simulink model "TD_ALBUQUERQUE_EVANGELISTA"  (R2020a)
settings: Solver=FixedStepAuto  StartTime=0.0  StopTime=tf  FixedStep=Ts  RelTol=1e-3
values from neighbouring files (symbols this model uses):
  alphas = [0 ; pi/2; 0  ; pi/2; -pi/2; pi/2;  0]    [Matlab_model.m]    (also in init.m)
  ds = [0 ;   0 ; d3 ;  0  ;    0 ;   0 ;  0]    [Matlab_model.m]    (also in init.m)
  Gravity = [0;0;-9.81]    [init.m]
  Gs = [G1,G2,G3,G4,G5,G6]    [Matlab_model.m]    (also in init.m)
  I = eye(3)    [Matlab_model.m]    (also in init.m = cat(3, I1,I2,I3,I4,I5,I6))
  Jm = 10e-6.*[1;1;1;1;1;1]    [Matlab_model.m]    (also in init.m)
  Kd = [1000;1000;500;100;100;500]    [init.m]
  Kp = [5000;8000;5500;800;5500;2500]    [init.m]
  m = [m1;m2;m3;m4;m5;m6]    [Matlab_model.m]    (also in init.m)
  Offset = [0; 0; pi/2; 0; 0; 0]    [init.m]
  q_dot_i = [0;0;0;0;0;0]    [Matlab_model.m]    (also in init.m)
  qdf = [0;1;0;0;0;0]    [Matlab_model.m]    (also in init.m)
  qdi = [-1;0;-1;-1;-1;-1]    [Matlab_model.m]    (also in init.m)
  red = [100;100;100;70;70;70]    [Matlab_model.m]    (also in init.m)
  rs = [r1;   0 ; 0  ; r4  ;    0 ;   0 ; rE]    [Matlab_model.m]    (also in init.m)
settings Model: OrderedModelArguments=off  Creator=vitor  LastModifiedBy=joaov

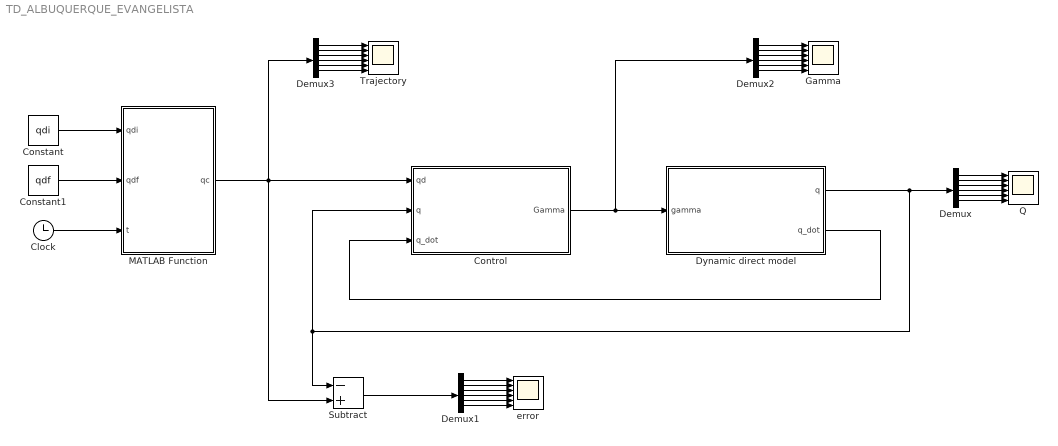
== system TD_ALBUQUERQUE_EVANGELISTA ==
  Clock : Clock
  Constant : Constant  Value=qdi
  Constant1 : Constant  Value=qdf
  Control : Subsystem
  Demux{,1..3} (4 alike) : Demux  Outputs=6
  Dynamic direct model : Subsystem
  Gamma : Scope  NumInputPorts=6
  MATLAB Function : MATLAB Function  TreatAsAtomicUnit=on
  Q : Scope  NumInputPorts=6
  Subtract : Sum  Inputs=-+
  Trajectory : Scope  NumInputPorts=6
  error : Scope  NumInputPorts=6
  wires:
  Demux/2 -> Q/2
  Demux/3 -> Q/3
  Demux/4 -> Q/4
  Demux/5 -> Q/5
  Demux/6 -> Q/6
  Dynamic direct model/1(q) -> Demux/1, Subtract/1, Control/2(q)
  Constant/1 -> MATLAB Function/1(qdi)
  Constant1/1 -> MATLAB Function/2(qdf)
  Clock/1 -> MATLAB Function/3(t)
  Demux1/5 -> error/5
  Demux1/2 -> error/2
  Demux1/3 -> error/3
  Demux1/6 -> error/6
  Demux1/4 -> error/4
  Demux1/1 -> error/1
  Subtract/1 -> Demux1/1
  Demux2/4 -> Gamma/4
  Demux2/2 -> Gamma/2
  Demux2/1 -> Gamma/1
  Demux2/5 -> Gamma/5
  Demux2/3 -> Gamma/3
  Demux2/6 -> Gamma/6
  Demux3/5 -> Trajectory/5
  Demux3/2 -> Trajectory/2
  Demux3/3 -> Trajectory/3
  Demux3/1 -> Trajectory/1
  Demux3/6 -> Trajectory/6
  Demux3/4 -> Trajectory/4
  MATLAB Function/1(qc) -> Subtract/2, Control/1(qd), Demux3/1
  Dynamic direct model/2(q_dot) -> Control/3(q_dot)
  Control/1(Gamma) -> Dynamic direct model/1(gamma), Demux2/1
  Demux/1 -> Q/1

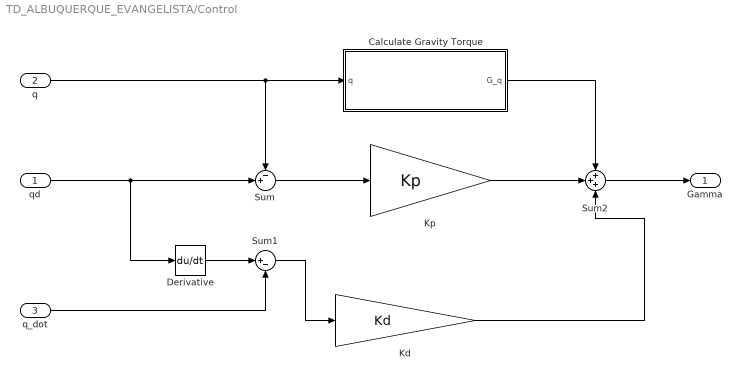
== system TD_ALBUQUERQUE_EVANGELISTA/Control ==
  qd : Inport
  q : Inport  Port=2
  q_dot : Inport  Port=3
  Calculate Gravity Torque : MATLAB Function  TreatAsAtomicUnit=on
  Derivative : Derivative
  Kd : Gain  Gain=Kd
  Kp : Gain  Gain=Kp
  Sum : Sum  Inputs=-+|
  Sum1 : Sum  Inputs=|+-
  Sum2 : Sum  Inputs=+++
  Gamma : Outport
  wires:
  Sum2/1 -> Gamma/1
  Kp/1 -> Sum2/2
  Sum/1 -> Kp/1
  qd/1 -> Sum/2, Derivative/1
  Calculate Gravity Torque/1(G_q) -> Sum2/1
  Kd/1 -> Sum2/3
  Sum1/1 -> Kd/1
  q/1 -> Sum/1, Calculate Gravity Torque/1(q)
  Derivative/1 -> Sum1/1
  q_dot/1 -> Sum1/2

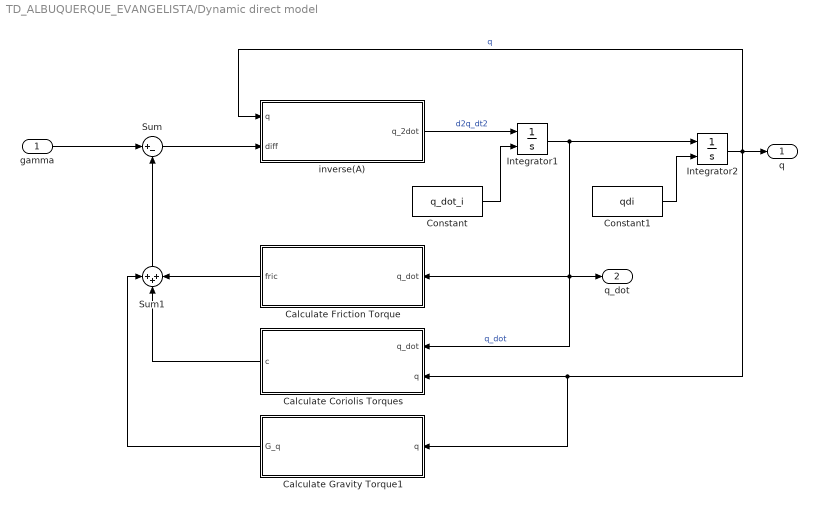
== system TD_ALBUQUERQUE_EVANGELISTA/Dynamic direct model ==
  gamma : Inport
  Calculate Coriolis Torques : MATLAB Function  TreatAsAtomicUnit=on
  Calculate Friction Torque : MATLAB Function  TreatAsAtomicUnit=on
  Calculate Gravity Torque1 : MATLAB Function  TreatAsAtomicUnit=on
  Constant : Constant  Value=q_dot_i
  Constant1 : Constant  Value=qdi
  Integrator1 : Integrator  InitialConditionSource=external
  Integrator2 : Integrator  InitialConditionSource=external
  Sum : Sum  Inputs=|+-
  Sum1 : Sum  Inputs=+++
  inverse(A) : MATLAB Function  TreatAsAtomicUnit=on
  q : Outport
  q_dot : Outport  Port=2
  wires:
  gamma/1 -> Sum/1
  Sum/1 -> inverse(A)/2(diff)
  inverse(A)/1(q_2dot) -> Integrator1/1  "d2q_dt2"
  Integrator1/1 -> Integrator2/1, q_dot/1, Calculate Coriolis Torques/1(q_dot), Calculate Friction Torque/1(q_dot)  "q_dot"
  Integrator2/1 -> Calculate Gravity Torque1/1(q), Calculate Coriolis Torques/2(q), q/1, inverse(A)/1(q)  "q"
  Calculate Coriolis Torques/1(c) -> Sum1/2
  Calculate Gravity Torque1/1(G_q) -> Sum1/1
  Calculate Friction Torque/1(fric) -> Sum1/3
  Sum1/1 -> Sum/2
  Constant/1 -> Integrator1/2
  Constant1/1 -> Integrator2/2

== matlab function TD_ALBUQUERQUE_EVANGELISTA/Dynamic direct model/Calculate Coriolis Torques ==
  data: q_dot input; q input; c output; I parameter; Gs parameter; Offset parameter
function c = ComputeCCTorques(q_dot,q,I,Gs,Offset)
    % Initialisation
    c=zeros(size(q));

    % Paramètres
    iI = I;
    x_G=Gs(1,:)';
    y_G=Gs(2,:)';
    z_G=Gs(3,:)';
    d3 = 0.7; 
    r1 = 0.5; r3=0.0 ; r4 = 0.2;
    alpha = [ 0 , pi/2 , 0 , pi/2 , -pi/2 , pi/2 ] ;
    alpha = [ 0 , pi/2 , 0 , pi/2 , -pi/2 , pi/2 ] ;
    theta = q + Offset;


    % Paramètres relatifs aux corps
    % Axe 1 %[0.80 0 0.05 ; 0 0.80 0 ; 0.05  0  0.10]
    XX1=0.80;
    XY1=0;
    XZ1=0.05;
    YY1=0.80;
    YZ1=0;
    ZZ1=0.10;

    M1=15;

    MX1=0*M1; %x_G1 = 0; y_G1 = 0; z_G1 = -0.25;
    MY1=0*M1;
    MZ1=-0.25*M1;

    % Axe 2 %[0.10  0  0.10; 0  1.50 0 ; 0.10  0  1.50]
    XX2=0.10;
    XY2=0;
    XZ2=0.10;
    YY2=1.50;
    YZ2=0;
    ZZ2=1.50;

    M2=10;

    MX2=0.35*M2; %x_G2 = 0.35; y_G2 = 0; z_G2 = 0;
    MY2=0*M2;
    MZ2=0*M2;

    % Axe 3 %[0.05 0 0 ; 0 0.01 0 ; 0 0 0.05]
    XX3=0.05;
    XY3=0;
    XZ3=0;
    YY3=0.01;
    YZ3=0;
    ZZ3=0.05;

    M3=1;

    MX3=0*M3; %x_G3 = 0; y_G3 = -0.1; z_G3 = 0;
    MY3=-0.1*M3;
    MZ3=0*M3;

    % Axe 4 %[0.50 0 0 ; 0 0.50 0 ; 0 0 0.05]
    XX4=0.50;
    XY4=0;
    XZ4=0;
    YY4=0.50;
    YZ4=0;
    ZZ4=0.05;

    M4=7;

    MX4=0*M4; %x_G4 = 0; y_G4 = 0; z_G4 = 0;
    MY4=0*M4;
    MZ4=0*M4;

    % Axe 5 %[0.01 0 0 ; 0 0.01 0 ; 0 0 0.01]
    XX5=0.01;
    XY5=0;
    XZ5=0;
    YY5=0.01;
    YZ5=0;
    ZZ5=0.01;

    M5=1;

    MX5=0*M5; %x_G5 = 0; y_G5 = 0; z_G5 = 0;
    MY5=0*M5; 
    MZ5=0*M5;

    % Axe 6 %[0.01 0 0 ; 0 0.01 0 ; 0 0 0.01]
    XX6=0.01;
    XY6=0;
    XZ6=0;
    YY6=0.01;
    YZ6=0;
    ZZ6=0.01;

    M6=0.5;

    MX6=0*M6; %x_G6 = 0; y_G6 = 0; z_G6 = 0;
    MY6=0*M6;
    MZ6=0*M6;

    % Valeurs angulaires
    t1=theta(1);
    t2=theta(2);
    t3=theta(3);
    t4=theta(4);
    t5=theta(5);
    t6=theta(6);

    C1 = cos(t1);
    S1 = sin(t1);
    C2 = cos(t2);
    S2 = sin(t2);
    C3 = cos(t3);
    S3 = sin(t3);
    C4 = cos(t4);
    S4 = sin(t4);
    C5 = cos(t5);
    S5 = sin(t5);
    C6 = cos(t6);
    S6 = sin(t6);

    % Vitesses articulaires
    QP1=q_dot(1);
    QP2=q_dot(2);
    QP3=q_dot(3);
    QP4=q_dot(4);
    QP5=q_dot(5);
    QP6=q_dot(6);
    
    % Paramètres regroupés
    XXR6 = XX6 - YY6;

    MR5 = M5 + M6;
    XXR5 = XX5 - YY5 + YY6;
    ZZR5 = YY6 + ZZ5;
    MYR5 = MY5 - MZ6;

    LamMS134 = 2*r4;
    LamM14 = r4^2;
    MR4 = M4 + MR5;
    XXR4 = XX4 - YY4 + YY5;
    ZZR4 = YY5 + ZZ4;
    MYR4 = MY4 + MZ5;

    LamMS133 = 2*r3;
    LamM13 = r3^2;
    LamM33 = -d3*r3;
    LamM43 = d3^2 + r3^2;
    LamM63 = d3^2;
    MR3 = M3 + MR4;
    XXR3 = LamM14*MR4 + LamMS134*MZ4 + XX3 - YY3 + YY4;
    ZZR3 = LamM14*MR4 + LamMS134*MZ4 + YY4 + ZZ3;
    MYR3 = -MR4*r4 + MY3 - MZ4;

    YYR2 = LamM43*MR3 + LamMS133*MZ3 + YY2 + YY3;
    MZR2 = MR3*r3 + MZ2 + MZ3;
    MR2 = M2 + MR3;
    XXR2 = LamM13*MR3 + LamMS133*MZ3 + XX2 + YY3 - YYR2;
    XZR2 = LamM33*MR3 - MZ3*d3 + XZ2;
    % ZZR2 = IA2 + LamM63*MR3 + ZZ2;
    ZZR2 = LamM63*MR3 + ZZ2;
    MXR2 = MR3*d3 + MX2;

    MR1 = M1 + MR2;
    % ZZR1 = IA1 + YYR2 + ZZ1;
    ZZR1 = YYR2 + ZZ1;

    IA1=0;
    IA2=0;
    IA3=0;
    IA4=0;
    IA5=0;
    IA6=0;

    FX6=0;
    FX5=0;
    FX4=0;
    FX3=0;
    FX2=0;
    FX1=0;
    FY6=0;
    FY5=0;
    FY4=0;
    FY3=0;
    FY2=0;
    FY1=0;
    FZ6=0;
    FZ5=0;
    FZ4=0;
    FZ3=0;
    FZ2=0;
    FZ1=0;
    CX6=0;
    CX5=0;
    CX4=0;
    CX3=0;
    CX2=0;
    CX1=0;
    CY6=0;
    CY5=0;
    CY4=0;
    CY3=0;
    CY2=0;
    CY1=0;
    CZ6=0;
    CZ5=0;
    CZ4=0;
    CZ3=0;
    CZ2=0;
    CZ1=0;
    FS1=0;
    FS2=0;
    FS3=0;
    FS4=0;
    FS5=0;
    FS6=0;
    FV1=0;
    FV2=0;
    FV3=0;
    FV4=0;
    FV5=0;
    FV6=0;


    % Calcul des couples de Coriolis et centrifuge
    
    G3=0; % Pour supprimer les termes de gravité

    DV61 = QP1^2;
    W12 = QP1*S2;
    W22 = C2*QP1;
    WP12 = QP2*W22;
    WP22 = -QP2*W12;
    DV12 = W12^2;
    DV22 = W12*W22;
    DV42 = W22^2;
    DV62 = QP2^2;
    U112 = -DV42 - DV62;
    U312 = -2*WP22;
    U222 = -DV12 - DV62;
    U322 = 2*WP12;
    U332 = -DV12 - DV42;
    VP12 = G3*S2;
    VP22 = C2*G3;
    W13 = C3*W12 + S3*W22;
    W23 = C3*W22 - S3*W12;
    W33 = QP2 + QP3;
    WP13 = C3*WP12 + QP3*W23 + S3*WP22;
    WP23 = C3*WP22 - QP3*W13 - S3*WP12;
    DV13 = W13^2;
    DV23 = W13*W23;
    DV33 = W13*W33;
    DV43 = W23^2;
    DV53 = W23*W33;
    DV63 = W33^2;
    U113 = -DV43 - DV63;
    U313 = DV33 - WP23;
    U223 = -DV13 - DV63;
    U323 = DV53 + WP13;
    U133 = DV33 + WP23;
    U233 = DV53 - WP13;
    U333 = -DV13 - DV43;
    VSP13 = U112*d3 + VP12;
    VSP23 = DV22*d3 + VP22;
    VSP33 = U312*d3 + U332*r3;
    VP13 = C3*VSP13 + S3*VSP23;
    VP23 = C3*VSP23 - S3*VSP13;
    W14 = C4*W13 + S4*W33;
    W24 = C4*W33 - S4*W13;
    W34 = QP4 - W23;
    WP14 = C4*WP13 + QP4*W24;
    WP24 = -QP4*W14 - S4*WP13;
    DV14 = W14^2;
    DV24 = W14*W24;
    DV34 = W14*W34;
    DV44 = W24^2;
    DV54 = W24*W34;
    DV64 = W34^2;
    U114 = -DV44 - DV64;
    U214 = DV24 - WP23;
    U314 = DV34 - WP24;
    U124 = DV24 + WP23;
    U224 = -DV14 - DV64;
    U324 = DV54 + WP14;
    U134 = DV34 + WP24;
    U234 = DV54 - WP14;
    U334 = -DV14 - DV44;
    VSP14 = -DV23*r4 + VP13;
    VSP24 = -U223*r4 + VP23;
    VSP34 = -U323*r4 + VSP33;
    VP14 = C4*VSP14 + S4*VSP34;
    VP24 = C4*VSP34 - S4*VSP14;
    W15 = C5*W14 - S5*W34;
    W25 = -C5*W34 - S5*W14;
    W35 = QP5 + W24;
    WP15 = C5*WP14 + QP5*W25 + S5*WP23;
    WP25 = C5*WP23 - QP5*W15 - S5*WP14;
    DV15 = W15^2;
    DV25 = W15*W25;
    DV35 = W15*W35;
    DV45 = W25^2;
    DV55 = W25*W35;
    DV65 = W35^2;
    U115 = -DV45 - DV65;
    U215 = DV25 + WP24;
    U315 = DV35 - WP25;
    U125 = DV25 - WP24;
    U225 = -DV15 - DV65;
    U325 = DV55 + WP15;
    U135 = DV35 + WP25;
    U235 = DV55 - WP15;
    U335 = -DV15 - DV45;
    VP15 = C5*VP14 + S5*VSP24;
    VP25 = C5*VSP24 - S5*VP14;
    W16 = C6*W15 + S6*W35;
    W26 = C6*W35 - S6*W15;
    W36 = QP6 - W25;
    WP16 = C6*WP15 + QP6*W26 + S6*WP24;
    WP26 = C6*WP24 - QP6*W16 - S6*WP15;
    DV16 = W16^2;
    DV26 = W16*W26;
    DV36 = W16*W36;
    DV46 = W26^2;
    DV56 = W26*W36;
    DV66 = W36^2;
    U116 = -DV46 - DV66;
    U216 = DV26 - WP25;
    U316 = DV36 - WP26;
    U126 = DV26 + WP25;
    U226 = -DV16 - DV66;
    U326 = DV56 + WP16;
    U136 = DV36 + WP26;
    U236 = DV56 - WP16;
    U336 = -DV16 - DV46;
    VP16 = C6*VP15 + S6*VP24;
    VP26 = C6*VP24 - S6*VP15;
    PSI31 = QP1*ZZR1;
    F12 = DV22*MY2 + MXR2*U112;
    F22 = DV22*MXR2 + MY2*U222;
    F32 = MXR2*U312 + MY2*U322;
    PSI12 = QP2*XZR2 + W12*XXR2 + W22*XY2;
    PSI22 = QP2*YZ2 + W12*XY2;
    PSI32 = QP2*ZZR2 + W12*XZR2 + W22*YZ2;
    No12 = -PSI22*QP2 + PSI32*W22 + WP12*XXR2 + WP22*XY2;
    No22 = PSI12*QP2 - PSI32*W12 + WP12*XY2;
    No32 = -PSI12*W22 + PSI22*W12 + WP12*XZR2 + WP22*YZ2;
    F13 = DV23*MYR3 + MX3*U113;
    F23 = DV23*MX3 + MYR3*U223;
    F33 = MX3*U313 + MYR3*U323;
    PSI13 = W13*XXR3 + W23*XY3 + W33*XZ3;
    PSI23 = W13*XY3 + W33*YZ3;
    PSI33 = W13*XZ3 + W23*YZ3 + W33*ZZR3;
    No13 = -PSI23*W33 + PSI33*W23 + WP13*XXR3 + WP23*XY3;
    No23 = PSI13*W33 - PSI33*W13 + WP13*XY3;
    No33 = -PSI13*W23 + PSI23*W13 + WP13*XZ3 + WP23*YZ3;
    F14 = MX4*U114 + MYR4*U124;
    F24 = MX4*U214 + MYR4*U224;
    F34 = MX4*U314 + MYR4*U324;
    PSI14 = W14*XXR4 + W24*XY4 + W34*XZ4;
    PSI24 = W14*XY4 + W34*YZ4;
    PSI34 = W14*XZ4 + W24*YZ4 + W34*ZZR4;
    No14 = -PSI24*W34 + PSI34*W24 + WP14*XXR4 - WP23*XZ4 + WP24*XY4;
    No24 = PSI14*W34 - PSI34*W14 + WP14*XY4 - WP23*YZ4;
    No34 = -PSI14*W24 + PSI24*W14 + WP14*XZ4 - WP23*ZZR4 + WP24*YZ4;
    F15 = MX5*U115 + MYR5*U125;
    F25 = MX5*U215 + MYR5*U225;
    F35 = MX5*U315 + MYR5*U325;
    PSI15 = W15*XXR5 + W25*XY5 + W35*XZ5;
    PSI25 = W15*XY5 + W35*YZ5;
    PSI35 = W15*XZ5 + W25*YZ5 + W35*ZZR5;
    No15 = -PSI25*W35 + PSI35*W25 + WP15*XXR5 + WP24*XZ5 + WP25*XY5;
    No25 = PSI15*W35 - PSI35*W15 + WP15*XY5 + WP24*YZ5;
    No35 = -PSI15*W25 + PSI25*W15 + WP15*XZ5 + WP24*ZZR5 + WP25*YZ5;
    F16 = MX6*U116 + MY6*U126;
    F26 = MX6*U216 + MY6*U226;
    F36 = MX6*U316 + MY6*U326;
    PSI16 = W16*XXR6 + W26*XY6 + W36*XZ6;
    PSI26 = W16*XY6 + W36*YZ6;
    PSI36 = W16*XZ6 + W26*YZ6 + W36*ZZ6;
    No16 = -PSI26*W36 + PSI36*W26 + WP16*XXR6 - WP25*XZ6 + WP26*XY6;
    No26 = PSI16*W36 - PSI36*W16 + WP16*XY6 - WP25*YZ6;
    No36 = -PSI16*W26 + PSI26*W16 + WP16*XZ6 - WP25*ZZ6 + WP26*YZ6;
    E16 = F16 + FX6;
    E26 = F26 + FY6;
    E36 = F36 + FZ6;
    N16 = CX6 - MY6*VP25 + No16;
    N26 = CY6 + MX6*VP25 + No26;
    N36 = CZ6 + MX6*VP26 - MY6*VP16 + No36;
    FDI16 = C6*E16 - E26*S6;
    FDI36 = C6*E26 + E16*S6;
    E15 = F15 + FDI16 + FX5;
    E25 = -E36 + F25 + FY5;
    E35 = F35 + FDI36 + FZ5;
    N15 = C6*N16 + CX5 + MYR5*VP24 - N26*S6 + No15;
    N25 = CY5 - MX5*VP24 - N36 + No25;
    N35 = C6*N26 + CZ5 + MX5*VP25 - MYR5*VP15 + N16*S6 + No35;
    FDI15 = C5*E15 - E25*S5;
    FDI35 = -C5*E25 - E15*S5;
    E14 = F14 + FDI15 + FX4;
    E24 = E35 + F24 + FY4;
    E34 = F34 + FDI35 + FZ4;
    N14 = C5*N15 + CX4 - MYR4*VSP24 - N25*S5 + No14;
    N24 = CY4 + MX4*VSP24 + N35 + No24;
    N34 = -C5*N25 + CZ4 + MX4*VP24 - MYR4*VP14 - N15*S5 + No34;
    FDI14 = C4*E14 - E24*S4;
    FDI34 = C4*E24 + E14*S4;
    E13 = F13 + FDI14 + FX3;
    E23 = -E34 + F23 + FY3;
    E33 = F33 + FDI34 + FZ3;
    N13 = C4*N14 + CX3 - FDI34*r4 + MYR3*VSP33 - N24*S4 + No13;
    N23 = CY3 - MX3*VSP33 - N34 + No23;
    N33 = C4*N24 + CZ3 + FDI14*r4 + MX3*VP23 - MYR3*VP13 + N14*S4 + No33;
    FDI13 = C3*E13 - E23*S3;
    FDI23 = C3*E23 + E13*S3;
    E12 = F12 + FDI13 + FX2;
    E22 = F22 + FDI23 + FY2;
    E32 = E33 + F32 + FZ2;
    N12 = C3*N13 + CX2 - FDI23*r3 - N23*S3 + No12;
    N22 = C3*N23 + CY2 - E33*d3 + FDI13*r3 + N13*S3 + No22;
    N32 = CZ2 + FDI23*d3 + MXR2*VP22 - MY2*VP12 + N33 + No32;
    FDI12 = C2*E12 - E22*S2;
    FDI32 = C2*E22 + E12*S2;
    E11 = FDI12 + FX1;
    E21 = -E32 + FY1;
    E31 = FDI32 + FZ1;
    N11 = C2*N12 + CX1 - N22*S2;
    N21 = CY1 - N32;
    N31 = C2*N22 + CZ1 + N12*S2;
   
    
    % Résultat
    c(1) = N31;
    c(2) = N32;
    c(3) = N33;
    c(4) = N34;
    c(5) = N35;
    c(6) = N36;
end

== matlab function TD_ALBUQUERQUE_EVANGELISTA/Dynamic direct model/inverse(A) ==
  data: q input; q_2dot output; diff input; alphas parameter; ds parameter; rs parameter; Gs parameter; m parameter; I parameter; red parameter; Jm parameter; Offset parameter
function q_2dot = invA(q, diff, alphas, ds, rs, Gs, m, I, red, Jm, Offset)
theta = q + Offset;
A_q = ComputeMatInert(theta,Gs,m,I,red,Jm,alphas,ds,rs);

q_2dot = pinv(A_q)*diff;


function A_q = ComputeMatInert(q,Gs,m,I,red,Jm,alphas,ds,rs)
% Exercise 13
% Computes the Inertia matrix of the manipulator A(q) in Rnxn
N = size(q,1);
A = zeros(N);
g = eye(4);

for i = 1:N
    g = g * TransformMatElem(alphas(i), ds(i), q(i), rs(i));
    
%     p0Oi = g(1:3,4);
    R0Oi = g(1:3,1:3);
    I_iOi = I(:,:,i);
    I_iGi = ComputeHuygens(I_iOi, m(i), [0;0;0], Gs(:,i));
    
    I_0Gi = R0Oi*I_iGi*R0Oi';
    
    [JvGi,JwGi] = ComputeJacGi(alphas, ds, q, rs, Gs, i);
    
    A = A + m(i).*(JvGi'*JvGi) + (JwGi'*I_0Gi*JwGi);
end

A_q = A + diag(Jm)*diag(red.^2);
end


function I_O = ComputeHuygens(I_G, m, O, G)
% Slide 166

O_G = G - O;

I_O = I_G + m*[O_G(2)*O_G(2)+O_G(3)*O_G(3), -O_G(1)*O_G(2), -O_G(1)*O_G(3);
                -O_G(1)*O_G(2), O_G(1)*O_G(1)+O_G(3)*O_G(3), -O_G(2)*O_G(3);
                -O_G(1)*O_G(3), -O_G(2)*O_G(3), O_G(1)*O_G(1)+O_G(2)*O_G(2)];
end


function g = TransformMatElem(a,d,t,r)
% Exercise 3.a (taken from slide 96)
% Computes the homogeneous transform matrix g between two successive frames
% Inputs: (alpha [rad] , d [m] , theta [rad] , r [m]) on MDH convention

% Expression: g = R_x(alpha)*Trans(x,di)*Rz(theta)*Trans(z,r)

% g = Rot_x(a)*Trans([d;0;0])*Rot_z(t)*Trans([0;0;r]);

% Alternative way of computation (faster computation)
g = [cos(t)       , -sin(t)      , 0      , d        ;
     cos(a)*sin(t), cos(a)*cos(t), -sin(a), -r*sin(a);
     sin(a)*sin(t), sin(a)*cos(t), cos(a) , r*cos(a) ;
     0            , 0            , 0      , 1        ];
end


function [JvGi,JwGi] = ComputeJacGi(alphas, ds, thetas, rs, Gs, n)
% Exercise 12
% Slide 168
% Returns the Jacobian matrix with respect center of mass of the body Ci and no longer the
% velocity of the origin of the robot's terminal frame

% Varignon formula : V(Gi) = V(OE) + w x OiGi
J0E = ComputeJac(alphas,ds,[thetas;0],rs);
[p0E,~] = ComputeDGM(alphas, ds, [thetas;0], rs);

JGi = zeros(size(J0E));
JGi_aux = zeros(size(J0E));
g = eye(4);

for i=1:n
    g = g * TransformMatElem(alphas(i),ds(i),thetas(i),rs(i));
    
    pOiGi_0 = g*[Gs(:,i);0];
    pOiGi_0 = pOiGi_0(1:3);
    
    Oe_Gi = g(1:3,4) + pOiGi_0 - p0E(1:3);
    Oe_Gi_matrix = vec_to_cross_prod(Oe_Gi);

    JGi_aux = [eye(3), -Oe_Gi_matrix; zeros(3), eye(3)]*J0E;
end

JGi(:,1:n) = JGi_aux(:,1:n);

JvGi = JGi(1:3,:);
JwGi = JGi(4:6,:);

end


function Jac = ComputeJac(a,d,t,r)
% Exercise 6 (taken from slide 107)
% Computes the Jacobian matrix of a tree with only revolute joints
% Inputs: (alphas [rad] , ds [m] , thetas [rad] , rs [m]) on MDH convention
%          with dimension N_joints + 1 x 1 (due to the end-effector)
% Output: J_0(q) (in R6xN)

N_joints = size(a,1) -1;
J = zeros(6,N_joints);
Zi = [0;0;1]; % The unit vector of the i-th joint given in frame Ri
g = eye(4);

[X0E,~] = ComputeDGM(a,d,t,r); % counting the end-effect
p0E = X0E(1:3);

for i = 1:N_joints
    g = g * TransformMatElem(a(i),d(i),t(i),r(i));
    R0i = g(1:3,1:3);
    p0i = g(1:3,4);
    
    pin = p0E - p0i;
    
    J(:,i) = [cross(R0i*Zi, pin);
                R0i*Zi]; % Since they are all revolute joints
end

Jac = J;
end


function [X, R0N] = ComputeDGM(alphas, ds, thetas, rs)
% Exercise 3.b (taken from slide 97)
% Computes the Direct geometric model g between two successive frames
% Inputs: (alphas [rad] , ds [m] , thetas [rad] , rs [m]) on MDH convention
%          each with dimension N x 1
% Output: X(q) = [px(q),py(q),pz(q),alpha(q),betta(q),gamma(q)]
%                                  (with the Euler angles convention)

[N_frames,~] = size(alphas);

% Computation of g0n recursively
g = eye(4);
for i = 1:N_frames
    g = g * TransformMatElem(alphas(i), ds(i), thetas(i), rs(i));
end

R0N = g(1:3,1:3);
euler_angs = get_euler_angles(R0N);
p0N = g(1:3,4);
X = [p0N; euler_angs];
end


function W = vec_to_cross_prod(w)
% Slide 60
% Computes the the skew-symmetric matrix associated 
% to the cross product of vectors w and u as follows w x u = Wu

W = [  0   , -w(3) ,  w(2);
      w(3) ,   0   , -w(1);
     -w(2) ,  w(1) ,   0  ];
end


function euler_angles = get_euler_angles(R)
% Slide 66 - Inverse relationship of euler angles
% Computes the Euler angles (alpha, betta, gamma) of a rotation matrix
% Input: Rotation matrix R (in SO(3))
g = atan2(R(3,1),R(3,2));
b = atan2(R(3,1)*sin(g) + R(3,2)*cos(g), R(3,3));
a = atan2(R(2,1)*cos(g) + R(2,2)*sin(g), R(1,1)*cos(g) - R(1,2)*sin(g));

euler_angles = [a;b;g];
end

end

== matlab function TD_ALBUQUERQUE_EVANGELISTA/Dynamic direct model/Calculate Friction Torque ==
  data: q_dot input; fric output; Fv parameter
function fric = ComputeFrictionTorque(q_dot,Fv)
% Exercise 17
% return the vector of joint torques produced by joint friction
% Friction model used:
% tau_f_i(q_dot_i) = diag(q_dot_i)*Fv_i for i = 1:6

fric = diag(q_dot)*Fv;
end

== matlab function TD_ALBUQUERQUE_EVANGELISTA/MATLAB Function ==
  data: qdi input; qc output; qdf input; t input; tf parameter
function qc = GenTraj(qdi, qdf, t, tf)
r = 10*(t/tf)^3 - 15*(t/tf)^4 + 6*(t/tf)^5;
D = qdf - qdi;
qc = qdi + r*D;

== matlab function TD_ALBUQUERQUE_EVANGELISTA/Control/Calculate Gravity Torque ==
  data: q input; G_q output; alphas parameter; ds parameter; rs parameter; Gs parameter; Gravity parameter; m parameter; Offset parameter
function G_q = ComputeGravTorque(q,alphas, ds, rs, Gs, Gravity, m, Offset)
% Exercise 15 (expression on TD2)
% Returns the vector of joint torques due
% to the gravity G(q) in R^6.
G = zeros(6,1);
N = length(q);

theta = q + Offset;

for j = 1:N
    [JvGi,~] = ComputeJacGi(alphas, ds, theta, rs, Gs, j);
    G = G - m(j).*(JvGi'*Gravity);
end

G_q = G;


function g = TransformMatElem(a,d,t,r)
% Exercise 3.a (taken from slide 96)
% Computes the homogeneous transform matrix g between two successive frames
% Inputs: (alpha [rad] , d [m] , theta [rad] , r [m]) on MDH convention

% Expression: g = R_x(alpha)*Trans(x,di)*Rz(theta)*Trans(z,r)

% g = Rot_x(a)*Trans([d;0;0])*Rot_z(t)*Trans([0;0;r]);

% Alternative way of computation (faster computation)
g = [cos(t)       , -sin(t)      , 0      , d        ;
     cos(a)*sin(t), cos(a)*cos(t), -sin(a), -r*sin(a);
     sin(a)*sin(t), sin(a)*cos(t), cos(a) , r*cos(a) ;
     0            , 0            , 0      , 1        ];
end

function [JvGi,JwGi] = ComputeJacGi(alphas, ds, thetas, rs, Gs, n)
% Exercise 12
% Slide 168
% Returns the Jacobian matrix with respect center of mass of the body Ci and no longer the
% velocity of the origin of the robot's terminal frame
% Inputs: (alphas [rad] , ds [m] , rs [m]) on MDH convention
%               each with dimension (N+1) x 1 with the End-effector's
%               parameters
%          thetas [rad] (in R nx1) --> joint-coordinates of the robot
%               (without the end-effector's parameter included)
%          Gs (in R 3xN) --> position of the barycenter of the bodies in
%               relation to their respective reference frames
%               i.e: OiGi in ref. frame Ri
%          i (in N*) between 1 and N --> index of the body to compute the
%               JacGi

J0E = ComputeJac(alphas,ds,[thetas;0],rs);
% p0E = Vector O0Oe in the 0 reference frame
[p0E,~] = ComputeDGM(alphas, ds, [thetas;0], rs); 

JGi = zeros(size(J0E));

% Getting the DGM until body i (g0i)
g = eye(4);
for i=1:n
    g = g * TransformMatElem(alphas(i),ds(i),thetas(i),rs(i));
end

O0Oi_0 = g(1:3,4); % Vector O0Oi in the 0 reference frame

pOiGi_0 = g*[Gs(:,n);0]; 
pOiGi_0 = pOiGi_0(1:3); % Vector OiGi in the 0 reference frame

Oe_Gi = O0Oi_0 + pOiGi_0 - p0E(1:3); % Vector OeGi in 0 reference frame
Oe_Gi_matrix = vec_to_cross_prod(Oe_Gi);

% Varignon formula : V(Gi) = V(OE) + w x OiGi (in matrix form) 
JGi_aux = [ eye(3)  , -Oe_Gi_matrix;
            zeros(3),      eye(3)  ]*J0E;

JGi(:,1:n) = JGi_aux(:,1:n);

JvGi = JGi(1:3,:);
JwGi = JGi(4:6,:);
end

function [X, R0N] = ComputeDGM(alphas, ds, thetas, rs)
% Exercise 3.b (taken from slide 97)
% Computes the Direct geometric model g between two successive frames
% Inputs: (alphas [rad] , ds [m] , thetas [rad] , rs [m]) on MDH convention
%          each with dimension N x 1
% Output: X(q) = [px(q),py(q),pz(q),alpha(q),betta(q),gamma(q)]
%                                  (with the Euler angles convention)

[N_frames,~] = size(alphas);

% Computation of g0n recursively
g = eye(4);
for i = 1:N_frames
    g = g * TransformMatElem(alphas(i), ds(i), thetas(i), rs(i));
end

R0N = g(1:3,1:3);
euler_angs = get_euler_angles(R0N);
p0N = g(1:3,4);
X = [p0N; euler_angs];
end

function Jac = ComputeJac(a,d,t,r)
% Exercise 6 (taken from slide 107)
% Computes the Jacobian matrix of a robot tree with only revolute joints
% Inputs: (alphas [rad] , ds [m] , thetas [rad] , rs [m]) on MDH convention
%          with dimension N_joints + 1 x 1 (due to the end-effector)
% Output: J_0(q) (in R6xN)

N_joints = size(a,1) -1;
J = zeros(6,N_joints);
Zi = [0;0;1]; % The unit vector of the i-th joint given in frame Ri
g = eye(4);

[X0E,~] = ComputeDGM(a,d,t,r); % counting the end-effect
p0E = X0E(1:3);

for i = 1:N_joints
    g = g * TransformMatElem(a(i),d(i),t(i),r(i));
    R0i = g(1:3,1:3);
    p0i = g(1:3,4);
    
    pin = p0E - p0i;
    
    J(:,i) = [cross(R0i*Zi, pin);
                R0i*Zi]; % Since they are all revolute joints
end

Jac = J;
end

function W = vec_to_cross_prod(w)
% Slide 60
% Computes the the skew-symmetric matrix associated 
% to the cross product of vectors w and u as follows w x u = Wu

W = [  0   , -w(3) ,  w(2);
      w(3) ,   0   , -w(1);
     -w(2) ,  w(1) ,   0  ];
end

function euler_angles = get_euler_angles(R)
% Slide 66 - Inverse relationship of euler angles
% Computes the Euler angles (alpha, betta, gamma) of a rotation matrix
% Input: Rotation matrix R (in SO(3))
g = atan2(R(3,1),R(3,2));
b = atan2(R(3,1)*sin(g) + R(3,2)*cos(g), R(3,3));
a = atan2(R(2,1)*cos(g) + R(2,2)*sin(g), R(1,1)*cos(g) - R(1,2)*sin(g));

euler_angles = [a;b;g];
end

end

== matlab function TD_ALBUQUERQUE_EVANGELISTA/Dynamic direct model/Calculate Gravity Torque1 ==
  data: q input; G_q output; alphas parameter; ds parameter; rs parameter; Gs parameter; Gravity parameter; m parameter; Offset parameter
function G_q = ComputeGravTorque(q,alphas, ds, rs, Gs, Gravity, m, Offset)
% Exercise 15 (expression on TD2)
% Returns the vector of joint torques due
% to the gravity G(q) in R^6.
G = zeros(6,1);
N = length(q);

theta = q + Offset;

for j = 1:N
    [JvGi,~] = ComputeJacGi(alphas, ds, theta, rs, Gs, j);
    G = G - m(j).*(JvGi'*Gravity);
end

G_q = G;


function g = TransformMatElem(a,d,t,r)
% Exercise 3.a (taken from slide 96)
% Computes the homogeneous transform matrix g between two successive frames
% Inputs: (alpha [rad] , d [m] , theta [rad] , r [m]) on MDH convention

% Expression: g = R_x(alpha)*Trans(x,di)*Rz(theta)*Trans(z,r)

% g = Rot_x(a)*Trans([d;0;0])*Rot_z(t)*Trans([0;0;r]);

% Alternative way of computation (faster computation)
g = [cos(t)       , -sin(t)      , 0      , d        ;
     cos(a)*sin(t), cos(a)*cos(t), -sin(a), -r*sin(a);
     sin(a)*sin(t), sin(a)*cos(t), cos(a) , r*cos(a) ;
     0            , 0            , 0      , 1        ];
end

function [JvGi,JwGi] = ComputeJacGi(alphas, ds, thetas, rs, Gs, n)
% Exercise 12
% Slide 168
% Returns the Jacobian matrix with respect center of mass of the body Ci and no longer the
% velocity of the origin of the robot's terminal frame
% Inputs: (alphas [rad] , ds [m] , rs [m]) on MDH convention
%               each with dimension (N+1) x 1 with the End-effector's
%               parameters
%          thetas [rad] (in R nx1) --> joint-coordinates of the robot
%               (without the end-effector's parameter included)
%          Gs (in R 3xN) --> position of the barycenter of the bodies in
%               relation to their respective reference frames
%               i.e: OiGi in ref. frame Ri
%          i (in N*) between 1 and N --> index of the body to compute the
%               JacGi

J0E = ComputeJac(alphas,ds,[thetas;0],rs);
% p0E = Vector O0Oe in the 0 reference frame
[p0E,~] = ComputeDGM(alphas, ds, [thetas;0], rs); 

JGi = zeros(size(J0E));

% Getting the DGM until body i (g0i)
g = eye(4);
for i=1:n
    g = g * TransformMatElem(alphas(i),ds(i),thetas(i),rs(i));
end

O0Oi_0 = g(1:3,4); % Vector O0Oi in the 0 reference frame

pOiGi_0 = g*[Gs(:,n);0]; 
pOiGi_0 = pOiGi_0(1:3); % Vector OiGi in the 0 reference frame

Oe_Gi = O0Oi_0 + pOiGi_0 - p0E(1:3); % Vector OeGi in 0 reference frame
Oe_Gi_matrix = vec_to_cross_prod(Oe_Gi);

% Varignon formula : V(Gi) = V(OE) + w x OiGi (in matrix form) 
JGi_aux = [ eye(3)  , -Oe_Gi_matrix;
            zeros(3),      eye(3)  ]*J0E;

JGi(:,1:n) = JGi_aux(:,1:n);

JvGi = JGi(1:3,:);
JwGi = JGi(4:6,:);
end

function [X, R0N] = ComputeDGM(alphas, ds, thetas, rs)
% Exercise 3.b (taken from slide 97)
% Computes the Direct geometric model g between two successive frames
% Inputs: (alphas [rad] , ds [m] , thetas [rad] , rs [m]) on MDH convention
%          each with dimension N x 1
% Output: X(q) = [px(q),py(q),pz(q),alpha(q),betta(q),gamma(q)]
%                                  (with the Euler angles convention)

[N_frames,~] = size(alphas);

% Computation of g0n recursively
g = eye(4);
for i = 1:N_frames
    g = g * TransformMatElem(alphas(i), ds(i), thetas(i), rs(i));
end

R0N = g(1:3,1:3);
euler_angs = get_euler_angles(R0N);
p0N = g(1:3,4);
X = [p0N; euler_angs];
end

function Jac = ComputeJac(a,d,t,r)
% Exercise 6 (taken from slide 107)
% Computes the Jacobian matrix of a robot tree with only revolute joints
% Inputs: (alphas [rad] , ds [m] , thetas [rad] , rs [m]) on MDH convention
%          with dimension N_joints + 1 x 1 (due to the end-effector)
% Output: J_0(q) (in R6xN)

N_joints = size(a,1) -1;
J = zeros(6,N_joints);
Zi = [0;0;1]; % The unit vector of the i-th joint given in frame Ri
g = eye(4);

[X0E,~] = ComputeDGM(a,d,t,r); % counting the end-effect
p0E = X0E(1:3);

for i = 1:N_joints
    g = g * TransformMatElem(a(i),d(i),t(i),r(i));
    R0i = g(1:3,1:3);
    p0i = g(1:3,4);
    
    pin = p0E - p0i;
    
    J(:,i) = [cross(R0i*Zi, pin);
                R0i*Zi]; % Since they are all revolute joints
end

Jac = J;
end

function W = vec_to_cross_prod(w)
% Slide 60
% Computes the the skew-symmetric matrix associated 
% to the cross product of vectors w and u as follows w x u = Wu

W = [  0   , -w(3) ,  w(2);
      w(3) ,   0   , -w(1);
     -w(2) ,  w(1) ,   0  ];
end

function euler_angles = get_euler_angles(R)
% Slide 66 - Inverse relationship of euler angles
% Computes the Euler angles (alpha, betta, gamma) of a rotation matrix
% Input: Rotation matrix R (in SO(3))
g = atan2(R(3,1),R(3,2));
b = atan2(R(3,1)*sin(g) + R(3,2)*cos(g), R(3,3));
a = atan2(R(2,1)*cos(g) + R(2,2)*sin(g), R(1,1)*cos(g) - R(1,2)*sin(g));

euler_angles = [a;b;g];
end

end
